simulink model "c_ep_approx_sim"  (R2024b)
settings: Solver=VariableStepAuto  StartTime=0.0  StopTime=10000  RelTol=1e-3
settings Model: Creator=merlin  LastModifiedBy=merlin

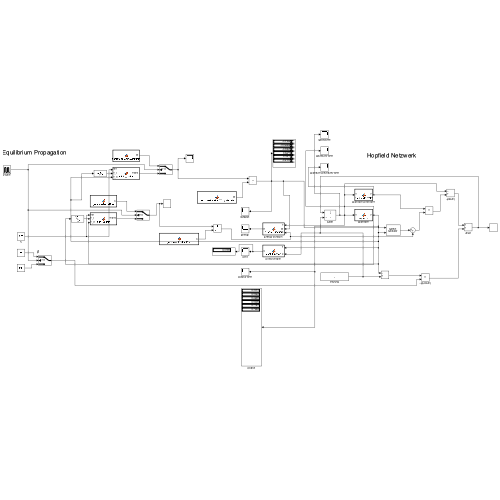
[thumbnail: Simulink's stored preview of the top-level diagram]
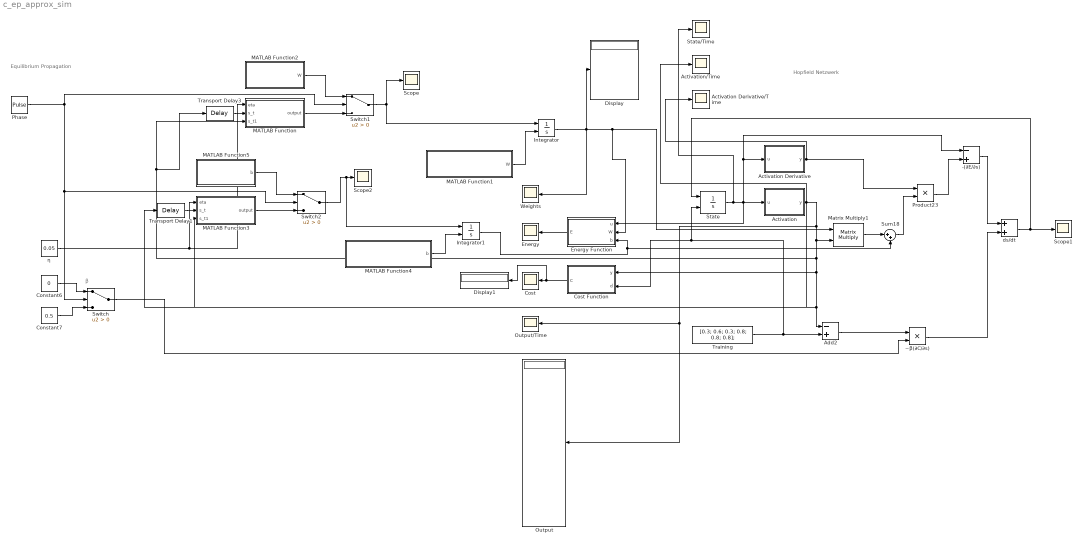
== system c_ep_approx_sim ==
  note: β
  note: Equilibrium Propagation
  note: Hopfield Netzwerk
  -(∂E/∂s) : Sum  Inputs=-+
  Activation : MATLAB Function  TreatAsAtomicUnit=on
  Activation Derivative : MATLAB Function  TreatAsAtomicUnit=on
  Activation Derivative/Time : Scope
  Activation/Time : Scope
  Add2 : Sum  Inputs=-+
  Constant6 : Constant  Value=0
  Constant7 : Constant  Value=0.5
  Cost : Scope
  Cost Function : MATLAB Function  TreatAsAtomicUnit=on
  Display : Display
  Display1 : Display
  Energy : Scope
  Energy Function : MATLAB Function  TreatAsAtomicUnit=on
  Integrator : Integrator  InitialConditionSource=external
  Integrator1 : Integrator  InitialConditionSource=external
  MATLAB Function : MATLAB Function  TreatAsAtomicUnit=on
  MATLAB Function1 : MATLAB Function  TreatAsAtomicUnit=on
  MATLAB Function2 : MATLAB Function  TreatAsAtomicUnit=on
  MATLAB Function3 : MATLAB Function  TreatAsAtomicUnit=on
  MATLAB Function4 : MATLAB Function  TreatAsAtomicUnit=on
  MATLAB Function5 : MATLAB Function  TreatAsAtomicUnit=on
  Matrix Multiply1 : Product  Multiplication=Matrix(*)
  Output : Display
  Output/Time : Scope
  Phase : DiscretePulseGenerator  PulseType=Time based  Period=20  PulseWidth=50
  Product23 : Product
  Scope : Scope
  Scope1 : Scope
  Scope2 : Scope
  State : Integrator  InitialConditionSource=external
  State/Time : Scope
  Sum18 : Sum  Inputs=|++
  Switch : Switch  Criteria=u2 > Threshold  SaturateOnIntegerOverflow=off  InputSameDT=off
  Switch1 : Switch  Criteria=u2 > Threshold  SaturateOnIntegerOverflow=off  InputSameDT=off
  Switch2 : Switch  Criteria=u2 > Threshold  SaturateOnIntegerOverflow=off  InputSameDT=off
  Training : Constant  Value=[0.3; 0.6; 0.3; 0.8; 0.8; 0.8];  VectorParams1D=off
  Transport Delay1 : TransportDelay
  Transport Delay3 : TransportDelay
  Weights : Scope
  ds/dt : Sum
  η : Constant  Value=0.05
  −β(∂C/∂s) : Product
  wires:
  Constant6/1 -> Switch/1
  Constant7/1 -> Switch/3
  Phase/1 -> Switch1/2, Switch/2, Switch2/2
  Product23/1 -> -(∂E/∂s)/2
  Energy Function/1(E) -> Energy/1
  −β(∂C/∂s)/1 -> ds/dt/2
  Cost Function/1(C) -> Display1/1, Cost/1
  ds/dt/1 -> Scope1/1, State/1
  Training/1 -> Cost Function/2(d), State/2, Add2/2
  -(∂E/∂s)/1 -> ds/dt/1
  Add2/1 -> −β(∂C/∂s)/1
  Sum18/1 -> Product23/2
  Matrix Multiply1/1 -> Sum18/1
  Activation Derivative/1(y) -> Activation Derivative/Time/1, Product23/1
  State/1 -> State/Time/1, Activation/1(u), Energy Function/1(u), -(∂E/∂s)/1, Activation Derivative/1(u)
  Activation/1(y) -> Transport Delay1/1, MATLAB Function/3(s_t1), Transport Delay3/1, MATLAB Function3/3(s_t1), Add2/1, Cost Function/1(y), Matrix Multiply1/2, Output/1, Output/Time/1, Activation/Time/1
  Switch/1 -> −β(∂C/∂s)/2
  Transport Delay3/1 -> MATLAB Function/2(s_t)
  η/1 -> MATLAB Function3/1(eta), MATLAB Function/1(eta)
  MATLAB Function1/1(W) -> Integrator/2
  Integrator/1 -> Energy Function/2(W), Matrix Multiply1/1, Display/1, Weights/1
  MATLAB Function/1(output) -> Switch1/3
  MATLAB Function2/1(W) -> Switch1/1
  Switch1/1 -> Integrator/1, Scope/1
  Transport Delay1/1 -> MATLAB Function3/2(s_t)
  MATLAB Function3/1(output) -> Switch2/3
  MATLAB Function5/1(b) -> Switch2/1
  Switch2/1 -> Integrator1/1, Scope2/1
  MATLAB Function4/1(b) -> Integrator1/2
  Integrator1/1 -> Sum18/2, Energy Function/3(b)

== matlab function c_ep_approx_sim/MATLAB Function1 ==
  data: W output
function W = generateRandomWeightMatrix()
n = 6;
W = randn(n);
W = (W + W') / 2;
W(1:n+1:end) = 0;
end

== matlab function c_ep_approx_sim/Energy Function ==
  data: u input; E output; W input; b input
function E = energy_function(u, W, b)
    rho = @(x) 1 ./ (1 + exp(-x));

    E = (1/2) * sum(u.^2) ...
        - (1/2) * sum(sum(W .* (rho(u) * rho(u)')))
        - sum(b .* rho(u));
end

== matlab function c_ep_approx_sim/MATLAB Function ==
  data: eta input; output output; s_t input; s_t1 input
function output = weight_update(eta, s_t, s_t1)
    output = eta * (s_t1 * s_t1' - s_t * s_t');
end

== matlab function c_ep_approx_sim/MATLAB Function2 ==
  data: W output
function W = generateZerosWeightMatrix()
n = 6;
W = zeros(n, n);
end

== matlab function c_ep_approx_sim/MATLAB Function3 ==
  data: eta input; output output; s_t input; s_t1 input
function output = bias_update(eta, s_t, s_t1)
    output = eta * (s_t1 - s_t);
end

== matlab function c_ep_approx_sim/MATLAB Function4 ==
  data: b output
function b = generateRandomBias()
% generateRandomBias generates an n x 1 vector of random bias values.
%
% Input:
%   n - number of neurons
%
% Output:
%   b - an n x 1 column vector of random bias values (drawn from a standard normal distribution)
%
% Example:
%   b = generateRandomBias(20);  % Returns a 20x1 vector of random biases.
n = 6;
b = randn(n, 1);
end

== matlab function c_ep_approx_sim/MATLAB Function5 ==
  data: b output
function b = generateZerosBias()
n = 6;
b = zeros(n, 1);
end

== matlab function c_ep_approx_sim/Activation Derivative ==
  data: u input; y output
function y = sigmoid_derivative(u)
% Activation Function: Logistic Function
% sigmoid = 1 ./ (1 + exp(-u));
% y = sigmoid .* (1 - sigmoid);

% Activation Function: Scaled Logistic Function
sigmoid = 1 ./ (1 + exp(-4 * u));
y = 4 .* sigmoid .* (1 - sigmoid);

% Activation Function: tanh
% y = 2 .* (1 - tanh(2 .* u).^2);

% Activation Function: ReLU
% y = double(u > 0);
end

== matlab function c_ep_approx_sim/Activation ==
  data: u input; y output
function y = sigmoid(u)
% Activation Function: Logistic Function
% y = 1 ./ (1 + exp(-u));

% Activation Function: Scaled Logistic Function
y = 1 ./ (1 + exp(-4 * u));

% Activation Function: tanh
% y = tanh(2 .* u);

% Activation Function: ReLU
% y = max(u, 0);
end

== matlab function c_ep_approx_sim/Cost Function ==
  data: y input; C output; d input
function C = cost_function(y, d)
    C = 0.5 * sum((y - d).^2);
end
